simulink model "taranis"  (Simulink 9.1)
settings: Solver=VariableStepAuto  StartTime=0.0  StopTime=inf  RelTol=1e-3
libraries: vrlib x1
settings Model: Creator=peter  LastModifiedBy=PSere
settings DataIOCC: SaveFormat=Dataset
settings OptimizationCC: LifeSpan=auto
settings DebuggingCC: UnderspecifiedInitializationDetection=Simplified  MergeDetectMultiDrivingBlocksExec=error  SFUnexpectedBacktrackingDiag=error  SFNoUnconditionalDefaultTransitionDiag=error  SFExecutionAtInitializationDiag=warning
settings HardwareCC: ProdBitPerPointer=64  ProdBitPerSizeT=64  ProdBitPerPtrDiffT=64  ProdLargestAtomicFloat=Float  ProdIntDivRoundTo=Zero  ProdEndianess=LittleEndian  ProdWordSize=64  ProdHWDeviceType=Intel->x86-64 (Windows64)
settings ModelReferenceCC: PropagateSignalLabelsOutOfModel=on
settings CodeAppCC: StateflowObjectComments=off
settings GRTTargetCC: TargetLangStandard=C99 (ISO)  CombineOutputUpdateFcns=on  GRTInterface=off
settings ConfigComp: CovMetricSettings=dwe  CovHtmlReporting=off  CovSaveCumulativeToWorkspaceVar=off  CovSaveSingleToWorkspaceVar=off  CovExternalEMLEnable=on

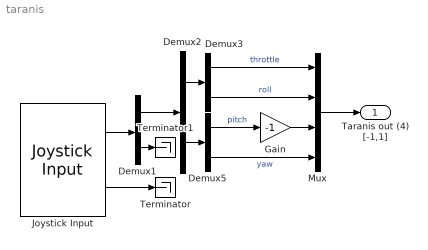
== system taranis ==
  Demux{1..3,5} (4 alike) : Demux  Outputs=2
  Gain : Gain  Gain=-1
  Joystick Input : vrlib/Joystick Input  joyid=1  adjustports=on  forcefeed=off
      settings: SourceProductBaseCode=VR
  Mux : Mux
  Terminator : Terminator
  Terminator1 : Terminator
  Taranis out (4) [-1,1] : Outport
  wires:
  Demux3/1 -> Mux/1  "throttle"
  Demux3/2 -> Mux/2  "roll"
  Demux5/1 -> Gain/1  "pitch"
  Demux5/2 -> Mux/4  "yaw"
  Mux/1 -> Taranis out (4) [-1,1]/1
  Demux2/1 -> Demux3/1
  Demux2/2 -> Demux5/1
  Demux1/1 -> Demux2/1
  Joystick Input/1 -> Demux1/1
  Demux1/2 -> Terminator1/1
  Joystick Input/2 -> Terminator/1
  Gain/1 -> Mux/3
